simulink model "sim_topic3"  (R2023b)
settings: Solver=FixedStepAuto  StartTime=0.0  StopTime=T_sim  FixedStep=dt_sim  RelTol=1e-3
undefined symbols (not defined in the file): den_Gd_tf_1, den_Gp_tf, Gd_ss_1, Gp_ss_1, num_Gd_tf_1, num_Gp_tf, T, x0
settings Model: Creator=user  LastModifiedBy=user

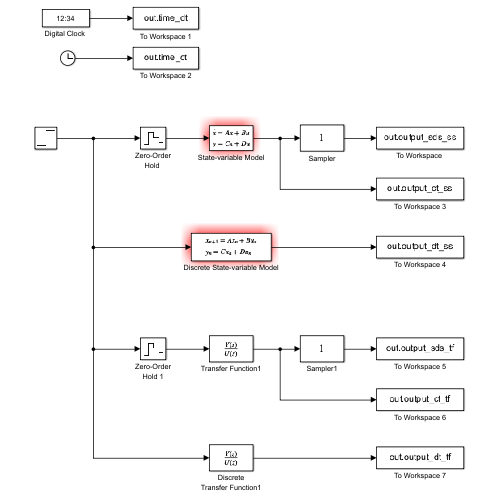
[thumbnail: Simulink's stored preview of the top-level diagram]
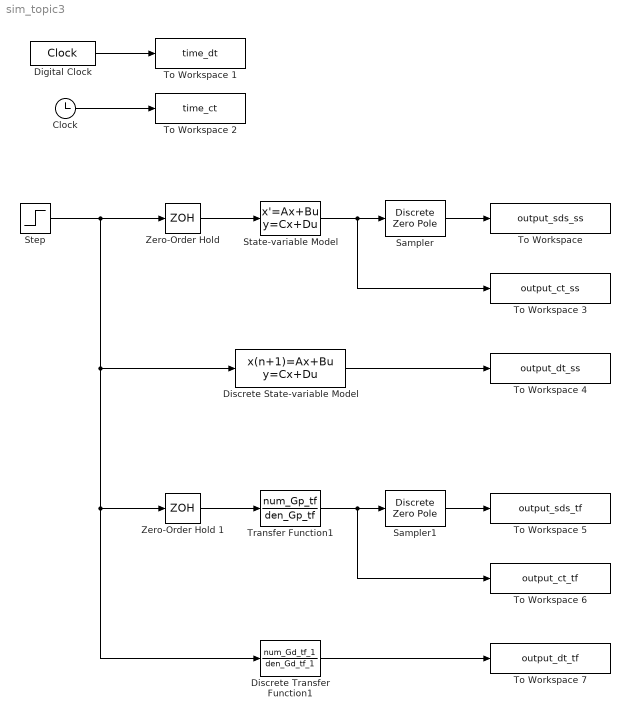
== system sim_topic3 ==
  Clock : Clock
  "Digital Clock " : DigitalClock  SampleTime=T
  Discrete Transfer Function1 : DiscreteTransferFcn  Numerator=num_Gd_tf_1  Denominator=den_Gd_tf_1
  Discrete State-variable Model : DiscreteStateSpace  A=Gd_ss_1.A  B=Gd_ss_1.B  C=Gd_ss_1.C  D=Gd_ss_1.D  InitialCondition=x0  SampleTime=T
  Sampler : DiscreteZeroPole  Zeros=[]  Poles=[]  Gain=1  SampleTime=T
  Sampler1 : DiscreteZeroPole  Zeros=[]  Poles=[]  Gain=1  SampleTime=T
  State-variable Model : StateSpace  A=Gp_ss_1.A  B=Gp_ss_1.B  C=Gp_ss_1.C  D=Gp_ss_1.D  InitialCondition=x0
  Step : Step  Time=0  SampleTime=T
  "To Workspace " : ToWorkspace  VariableName=output_sds_ss  SampleTime=T
  To Workspace 1 : ToWorkspace  VariableName=time_dt  SampleTime=T
  To Workspace 2 : ToWorkspace  VariableName=time_ct  SampleTime=-1
  To Workspace 3 : ToWorkspace  VariableName=output_ct_ss  SampleTime=-1
  To Workspace 4 : ToWorkspace  VariableName=output_dt_ss  SampleTime=T
  To Workspace 5 : ToWorkspace  VariableName=output_sds_tf  SampleTime=T
  To Workspace 6 : ToWorkspace  VariableName=output_ct_tf  SampleTime=-1
  To Workspace 7 : ToWorkspace  VariableName=output_dt_tf  SampleTime=T
  Transfer Function1 : TransferFcn  Numerator=num_Gp_tf  Denominator=den_Gp_tf
  "Zero-Order Hold " : ZeroOrderHold  SampleTime=-1
  Zero-Order Hold 1 : ZeroOrderHold  SampleTime=-1
  wires:
  Clock/1 -> To Workspace 2/1
  "Zero-Order Hold "/1 -> State-variable Model/1
  "Digital Clock "/1 -> To Workspace 1/1
  Sampler/1 -> "To Workspace "/1
  Discrete State-variable Model/1 -> To Workspace 4/1
  State-variable Model/1 -> To Workspace 3/1, Sampler/1
  Sampler1/1 -> To Workspace 5/1
  Discrete Transfer Function1/1 -> To Workspace 7/1
  Step/1 -> Discrete State-variable Model/1, Zero-Order Hold 1/1, Discrete Transfer Function1/1, "Zero-Order Hold "/1
  Transfer Function1/1 -> To Workspace 6/1, Sampler1/1
  Zero-Order Hold 1/1 -> Transfer Function1/1
